simulink subsystem "NoSuspension"  (R2022b)
settings: Solver=VariableStepAuto  StartTime=0.0  StopTime=10.0  RelTol=1e-3
settings Model: ModifiedByFormat=The MathWorks, Inc.  Creator=The MathWorks, Inc.  LastModifiedBy=The MathWorks, Inc.

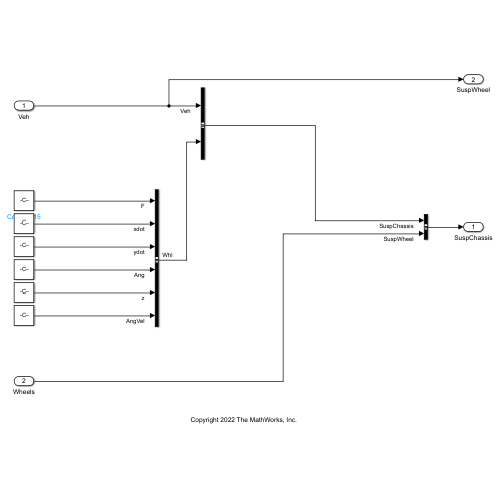
[thumbnail: Simulink's stored preview of the top-level diagram]
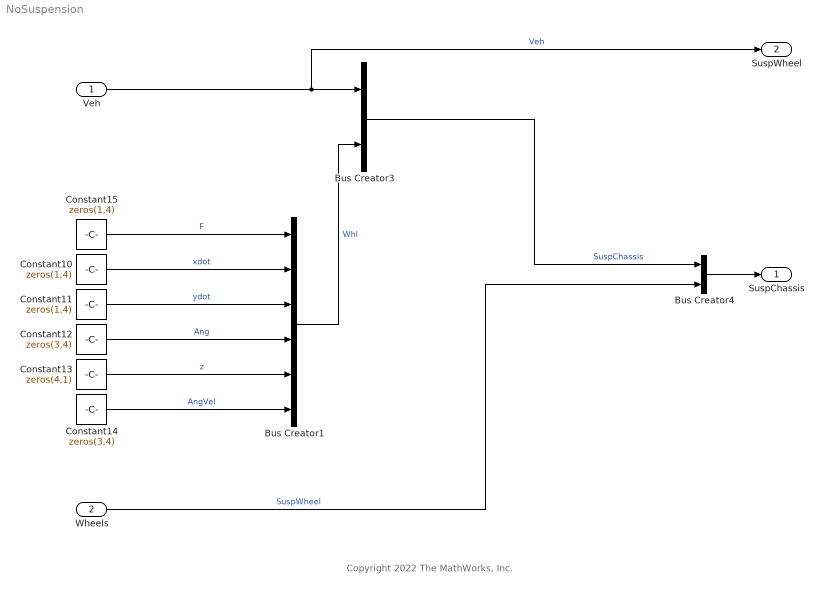
== system NoSuspension ==
  note: Copyright 2022 The MathWorks, Inc.
  Veh : Inport
  Wheels : Inport  Port=2
  Bus Creator1 : BusCreator  Inputs=6
  Bus Creator3 : BusCreator  Inputs=2
  Bus Creator4 : BusCreator  Inputs=2
  Constant10 : Constant  Value=zeros(1,4)  SampleTime=-1
  Constant11 : Constant  Value=zeros(1,4)  SampleTime=-1
  Constant12 : Constant  Value=zeros(3,4)  SampleTime=-1
  Constant13 : Constant  Value=zeros(4,1)  SampleTime=-1
  Constant14 : Constant  Value=zeros(3,4)  SampleTime=-1
  Constant15 : Constant  Value=zeros(1,4)  SampleTime=-1
  SuspChassis : Outport
  SuspWheel : Outport  Port=2
  wires:
  Bus Creator4/1 -> SuspChassis/1
  Veh/1 -> SuspWheel/1, Bus Creator3/1  "Veh"
  Bus Creator3/1 -> Bus Creator4/1  "SuspChassis"
  Wheels/1 -> Bus Creator4/2  "SuspWheel"
  Constant14/1 -> Bus Creator1/6  "AngVel"
  Constant13/1 -> Bus Creator1/5  "z"
  Constant10/1 -> Bus Creator1/2  "xdot"
  Bus Creator1/1 -> Bus Creator3/2  "Whl"
  Constant12/1 -> Bus Creator1/4  "Ang"
  Constant11/1 -> Bus Creator1/3  "ydot"
  Constant15/1 -> Bus Creator1/1  "F"
